simulink model "rf_thickener_open_loop"  (R2017a)
settings: Solver=VariableStepAuto  StartTime=0.0  StopTime=simTime  RelTol=1e-3  EnableMultiTasking=on
values from neighbouring files (symbols this model uses):
  addICInSimulation = zeros(1,5)    [OLD_compare_rf_thickener.m]    (also in OLD_compare_rf_thickener_PRBS.m; bogey.m = ones(1,5); compare_predictors.m = ones(1,5); compare_rf_thickener_RealData.m = ones(1,5))
  D0 = [325.1 0.3143 0.356]    [OLD_compare_rf_thickener.m]    (also in OLD_compare_rf_thickener_PRBS.m = [326.419 0.3 0.356]; bogey.m = [326.3733 0.3143 0.356]; compare_predictors.m = [326.3733 0.3143 0.356]; compare_rf_thickener_RealData.m = [326.3733 0.3143 0.356])
  Dt = 1    [OLD_compare_rf_thickener.m]    (also in OLD_compare_rf_thickener_PRBS.m; bogey.m; compare_predictors.m; compare_rf_thickener_RealData.m)
  m = length(MachineLearningData.MV)    [compare_predictors.m]    (also in compare_rf_thickener_RealData.m)
  make = makeMatrix(m,:)    [OLD_compare_rf_thickener.m]    (also in OLD_compare_rf_thickener_PRBS.m = makeMatrix(iterationSim,:); bogey.m = makeMatrix(iterationsSim,:); compare_predictors.m = makeStepMatrix(simIter,:); compare_rf_thickener_RealData.m = makeStepMatrix(simIter,:))
  nPredictors = [10 10 9 9]    [OLD_compare_rf_thickener.m]    (also in OLD_compare_rf_thickener_PRBS.m = [10 10 10 10])
  nTrees = [100 100 100 100]    [OLD_compare_rf_thickener.m]    (also in OLD_compare_rf_thickener_PRBS.m)
  tau_R = 10*groupBy    (= 600)    [OLD_compare_rf_thickener.m]    (also in OLD_compare_rf_thickener_PRBS.m = 300; bogey.m = 300; compare_predictors.m = 5; compare_rf_thickener_RealData.m = 300)
  U0 = [111 26]    [OLD_compare_rf_thickener.m]    (also in OLD_compare_rf_thickener_PRBS.m = [113.8675 25.715]; bogey.m = [114.8275 26.0152]; compare_predictors.m = [114.8275 26.0152]; compare_rf_thickener_RealData.m = [114.8275 26.0152])
undefined symbols (not defined in the file or in its folder): A, a1, a2, a3, B, b0, b1, b2, b3, b4, c0, c1, Cdata, Cz, Ddata, DiscIntNeverNeededParam, Dz, jf, kappa, L, lambda, mu, N, n_rz, na, nb, nc, phi0, phi_c, phi_f, rho_f, rho_s, theta, u10, u20, u30, v_max, w0, y, Z
settings Model: ExtModeTrigDuration=100  Creator=pablo  LastModifiedBy=Felipe
settings DataIOCC: SaveOutput=off  StateSaveName=tmp_raccel_xout  SignalLoggingName=tmp_raccel_logsout
settings OptimizationCC: EfficientMapNaN2IntZero=off  LifeSpan=inf
settings DebuggingCC: SFUnexpectedBacktrackingDiag=warning  SFNoUnconditionalDefaultTransitionDiag=warning  SFExecutionAtInitializationDiag=none
settings HardwareCC: TargetBitPerPointer=64  TargetBitPerSizeT=64  TargetBitPerPtrDiffT=64  TargetLongLongMode=on  TargetIntDivRoundTo=Zero  TargetEndianess=LittleEndian  TargetWordSize=64  TargetHWDeviceType=MATLAB Host  ProdEqTarget=off
settings RTWCC: SystemTargetFile=raccel.tlc  TemplateMakefile=raccel_default_tmf  RTWVerbose=off  RTWUseSimCustomCode=on
settings CodeAppCC: GenerateComments=off  MaxIdLength=128  MangleLength=10  SimulinkBlockComments=off
settings RaccelTargetCC: GeneratePreprocessorConditionals=Use local settings  ERTFirstTimeCompliant=off  MultiInstanceERTCode=off  ENABLE_SLEXEC_SSBRIDGE=0  RTWCAPIParams=on
settings ConfigComp: CovMetricSettings=dw  CovHtmlReporting=on  CovSaveCumulativeToWorkspaceVar=on  CovSaveSingleToWorkspaceVar=on  CovExternalEMLEnable=off

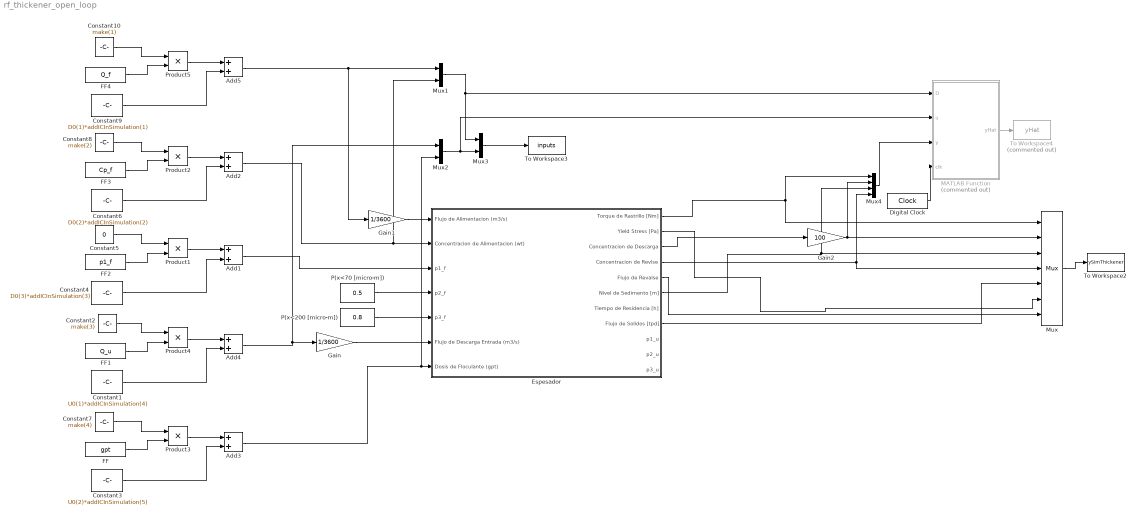
== system rf_thickener_open_loop ==
  Add{1..5} (5 alike) : Sum
  Constant1 : Constant  Value=U0(1)*addICInSimulation(4)
  Constant10 : Constant  Value=make(1)
  Constant2 : Constant  Value=make(3)
  Constant3 : Constant  Value=U0(2)*addICInSimulation(5)
  Constant4 : Constant  Value=D0(3)*addICInSimulation(3)
  Constant5 : Constant  Value=0
  Constant6 : Constant  Value=D0(2)*addICInSimulation(2)
  Constant7 : Constant  Value=make(4)
  Constant8 : Constant  Value=make(2)
  Constant9 : Constant  Value=D0(1)*addICInSimulation(1)
  Digital Clock : DigitalClock
  Espesador : Subsystem
  FF : FromWorkspace  VariableName=gpt  SampleTime=Dt
  FF1 : FromWorkspace  VariableName=Q_u  SampleTime=Dt
  FF2 : FromWorkspace  VariableName=p1_f  SampleTime=Dt
  FF3 : FromWorkspace  VariableName=Cp_f  SampleTime=Dt
  FF4 : FromWorkspace  VariableName=Q_f  SampleTime=Dt
  Gain : Gain  Gain=1/3600
  Gain1 : Gain  Gain=1/3600
  Gain2 : Gain  Gain=100
  MATLAB Function : MATLAB Function  Commented=on  TreatAsAtomicUnit=on
  Mux : Mux  Inputs=7
  Mux1 : Mux  Inputs=2
  Mux2 : Mux  Inputs=2
  Mux3 : Mux  Inputs=2
  Mux4 : Mux
  P(x<200 [micro-m]) : Constant  Value=0.8
  P(x<70 [micro-m]) : Constant  Value=0.5
  Product{1..5} (5 alike) : Product
  To Workspace2 : ToWorkspace  VariableName=ySimThickener  SaveFormat=Structure With Time  SampleTime=-1
  To Workspace3 : ToWorkspace  VariableName=inputs  SaveFormat=Structure With Time  SampleTime=-1
  To Workspace4 : ToWorkspace  Commented=on  VariableName=yHat  SaveFormat=Structure With Time  SampleTime=-1
  wires:
  P(x<200 [micro-m])/1 -> Espesador/5(p3_f)
  P(x<70 [micro-m])/1 -> Espesador/4(p2_f)
  FF/1 -> Product3/2
  Gain/1 -> Espesador/6(Flujo de Descarga Entrada (m3/s))
  Espesador/8(Flujo de Solidos [tpd]) -> Mux/5
  Espesador/2(Yield Stress [Pa]) -> Mux/6
  Espesador/5(Flujo de Revalse) -> Mux/7
  Mux/1 -> To Workspace2/1
  Constant7/1 -> Product3/1
  Product3/1 -> Add3/1
  Constant3/1 -> Add3/2
  Add3/1 -> Mux2/2, Espesador/7(Dosis de Floculante (gpt))
  Product4/1 -> Add4/1
  FF1/1 -> Product4/2
  Constant1/1 -> Add4/2
  Constant2/1 -> Product4/1
  Product1/1 -> Add1/1
  FF2/1 -> Product1/2
  Add1/1 -> Espesador/3(p1_f)
  Constant4/1 -> Add1/2
  Constant5/1 -> Product1/1
  Product2/1 -> Add2/1
  FF3/1 -> Product2/2
  Add2/1 -> Mux1/2, Espesador/2(Concentracion de Alimentacion (wt))
  Constant6/1 -> Add2/2
  Constant8/1 -> Product2/1
  Product5/1 -> Add5/1
  Constant10/1 -> Product5/1
  FF4/1 -> Product5/2
  Add5/1 -> Mux1/1, Gain1/1
  Constant9/1 -> Add5/2
  Add4/1 -> Mux2/1, Gain/1
  Mux3/1 -> To Workspace3/1
  Mux2/1 -> MATLAB Function/2(u), Mux3/2
  Mux1/1 -> Mux3/1, MATLAB Function/1(D)
  Digital Clock/1 -> MATLAB Function/4(clk)
  Mux4/1 -> MATLAB Function/3(y)
  MATLAB Function/1(yHat) -> To Workspace4/1
  Gain1/1 -> Espesador/1(Flujo de Alimentacion (m3/s))
  Espesador/1(Torque de Rastrillo [Nm]) -> Mux4/1, Mux/1
  Espesador/6(Nivel de Sedimento [m]) -> Mux/3, Mux4/3
  Espesador/4(Concentracion de Revlse) -> Mux/4, Mux4/4
  Espesador/3(Concentracion de Descarga) -> Gain2/1
  Gain2/1 -> Mux4/2, Mux/2

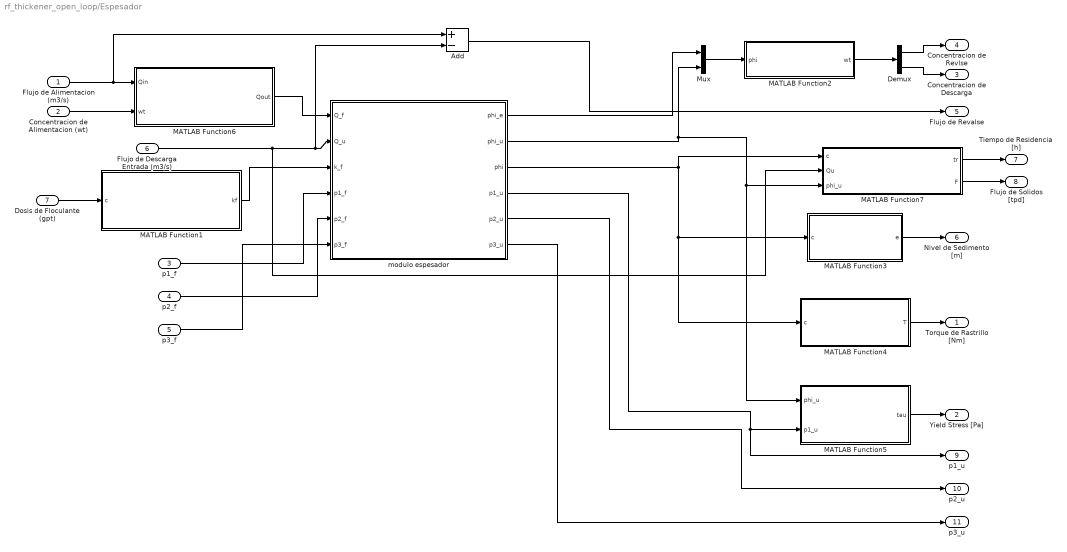
== system rf_thickener_open_loop/Espesador ==
  Flujo de Alimentacion (m3/s) : Inport
  Concentracion de Alimentacion (wt) : Inport  Port=2
  p1_f : Inport  Port=3
  p2_f : Inport  Port=4
  p3_f : Inport  Port=5
  Flujo de Descarga Entrada (m3/s) : Inport  Port=6
  Dosis de Floculante (gpt) : Inport  Port=7
  Add : Sum  Inputs=+-
  Demux : Demux  Outputs=2
  MATLAB Function1 : MATLAB Function  TreatAsAtomicUnit=on
  MATLAB Function2 : MATLAB Function  TreatAsAtomicUnit=on
  MATLAB Function3 : MATLAB Function  TreatAsAtomicUnit=on
  MATLAB Function4 : MATLAB Function  TreatAsAtomicUnit=on
  MATLAB Function5 : MATLAB Function  TreatAsAtomicUnit=on
  MATLAB Function6 : MATLAB Function  TreatAsAtomicUnit=on
  MATLAB Function7 : MATLAB Function  TreatAsAtomicUnit=on
  Mux : Mux  Inputs=2
  modulo espesador : Subsystem
  Torque de Rastrillo [Nm] : Outport
  Yield Stress [Pa] : Outport  Port=2
  Concentracion de Descarga : Outport  Port=3
  Concentracion de Revlse : Outport  Port=4
  Flujo de Revalse : Outport  Port=5
  Nivel de Sedimento [m] : Outport  Port=6
  Tiempo de Residencia [h] : Outport  Port=7
  Flujo de Solidos [tpd] : Outport  Port=8
  "p1_u " : Outport  Port=9
  "p2_u " : Outport  Port=10
  p3_u : Outport  Port=11
  wires:
  MATLAB Function3/1(e) -> Nivel de Sedimento [m]/1
  MATLAB Function4/1(T) -> Torque de Rastrillo [Nm]/1
  MATLAB Function5/1(tau) -> Yield Stress [Pa]/1
  Dosis de Floculante (gpt)/1 -> MATLAB Function1/1(c)
  Flujo de Descarga Entrada (m3/s)/1 -> MATLAB Function7/2(Qu), Add/2, modulo espesador/2(Q_u)
  MATLAB Function1/1(kf) -> modulo espesador/3(k_f)
  modulo espesador/1(phi_e) -> Mux/1
  modulo espesador/2(phi_u) -> MATLAB Function7/3(phi_u), MATLAB Function5/1(phi_u), Mux/2
  modulo espesador/5(p2_u) -> "p2_u "/1
  modulo espesador/3(phi) -> MATLAB Function7/1(c), MATLAB Function3/1(c), MATLAB Function4/1(c)
  p1_f/1 -> modulo espesador/4(p1_f)
  p2_f/1 -> modulo espesador/5("p2_f ")
  modulo espesador/4(p1_u) -> "p1_u "/1, MATLAB Function5/2(p1_u)
  Mux/1 -> MATLAB Function2/1(phi)
  MATLAB Function2/1(wt) -> Demux/1
  Demux/1 -> Concentracion de Revlse/1
  Demux/2 -> Concentracion de Descarga/1
  p3_f/1 -> modulo espesador/6(p3_f)
  modulo espesador/6(p3_u) -> p3_u/1
  MATLAB Function6/1(Qout) -> modulo espesador/1(Q_f)
  Flujo de Alimentacion (m3/s)/1 -> Add/1, MATLAB Function6/1(Qin)
  Concentracion de Alimentacion (wt)/1 -> MATLAB Function6/2(wt)
  MATLAB Function7/1(tr) -> Tiempo de Residencia [h]/1
  MATLAB Function7/2(F) -> Flujo de Solidos [tpd]/1
  Add/1 -> Flujo de Revalse/1

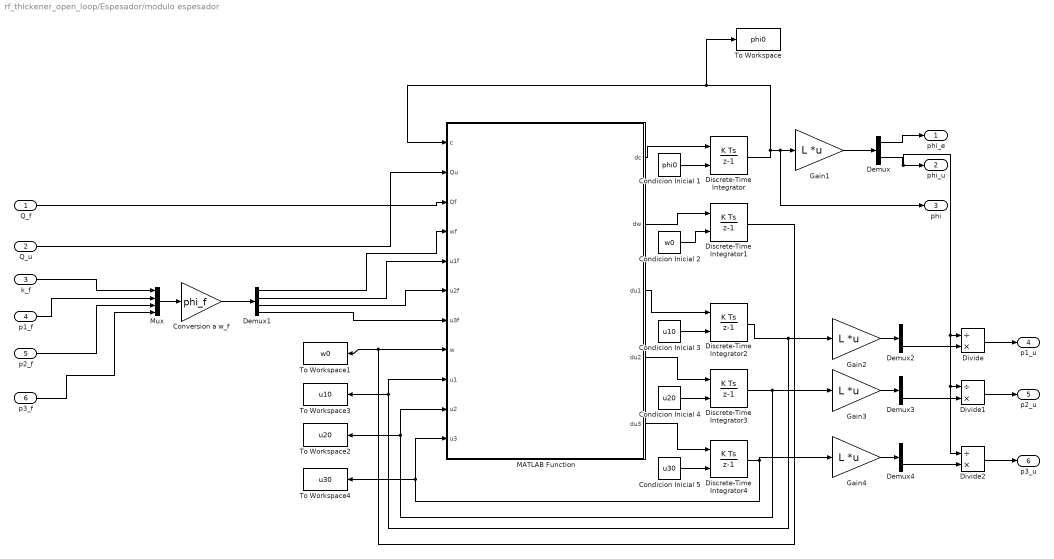
== system rf_thickener_open_loop/Espesador/modulo espesador ==
  Q_f : Inport
  Q_u : Inport  Port=2
  k_f : Inport  Port=3
  p1_f : Inport  Port=4
  "p2_f " : Inport  Port=5
  p3_f : Inport  Port=6
  Condicion Inicial 1 : Constant  Value=phi0
  Condicion Inicial 2 : Constant  Value=w0
  Condicion Inicial 3 : Constant  Value=u10
  Condicion Inicial 4 : Constant  Value=u20
  Condicion Inicial 5 : Constant  Value=u30
  Conversion a w_f : Gain  Gain=phi_f
  Demux{,2..4} (4 alike) : Demux  Outputs=2
  Demux1 : Demux
  Discrete-Time Integrator{,1..4} (5 alike) : DiscreteIntegrator  InitialConditionSource=external  InitialConditionSetting=State (most efficient)  SampleTime=Dt  ICPrevOutput=DiscIntNeverNeededParam  ICPrevScaledInput=DiscIntNeverNeededParam
  Divide : Product  Inputs=/*
  Divide1 : Product  Inputs=/*
  Divide2 : Product  Inputs=/*
  Gain{1..4} (4 alike) : Gain  Gain=L  Multiplication=Matrix(K*u) (u vector)
  MATLAB Function : MATLAB Function  TreatAsAtomicUnit=on
  Mux : Mux
  To Workspace : ToWorkspace  VariableName=phi0  SampleTime=-1
      settings: MaxDataPoints=1
  To Workspace1 : ToWorkspace  VariableName=w0  SampleTime=-1
      settings: MaxDataPoints=1
  To Workspace2 : ToWorkspace  VariableName=u20  SampleTime=-1
      settings: MaxDataPoints=1
  To Workspace3 : ToWorkspace  VariableName=u10  SampleTime=-1
      settings: MaxDataPoints=1
  To Workspace4 : ToWorkspace  VariableName=u30  SampleTime=-1
      settings: MaxDataPoints=1
  phi_e : Outport
  phi_u : Outport  Port=2
  phi : Outport  Port=3
  p1_u : Outport  Port=4
  p2_u : Outport  Port=5
  p3_u : Outport  Port=6
  wires:
  Discrete-Time Integrator/1 -> MATLAB Function/1(c), To Workspace/1, phi/1, Gain1/1
  Gain1/1 -> Demux/1
  Demux/1 -> phi_e/1
  Demux/2 -> Divide2/1, Divide1/1, Divide/1, phi_u/1
  MATLAB Function/1(dc) -> Discrete-Time Integrator/1
  Condicion Inicial 1/1 -> Discrete-Time Integrator/2
  Condicion Inicial 2/1 -> Discrete-Time Integrator1/2
  MATLAB Function/2(dw) -> Discrete-Time Integrator1/1
  Discrete-Time Integrator1/1 -> MATLAB Function/8(w), To Workspace1/1
  Q_f/1 -> MATLAB Function/3(Qf)
  Q_u/1 -> MATLAB Function/2(Qu)
  "p2_f "/1 -> Mux/3
  Mux/1 -> Conversion a w_f/1
  Conversion a w_f/1 -> Demux1/1
  Demux1/1 -> MATLAB Function/4(wf)
  Demux1/2 -> MATLAB Function/5(u1f)
  Demux1/3 -> MATLAB Function/6(u2f)
  Demux1/4 -> MATLAB Function/7(u3f)
  p3_f/1 -> Mux/4
  p1_f/1 -> Mux/2
  k_f/1 -> Mux/1
  Condicion Inicial 5/1 -> Discrete-Time Integrator4/2
  Condicion Inicial 4/1 -> Discrete-Time Integrator3/2
  MATLAB Function/5(du3) -> Discrete-Time Integrator4/1
  Discrete-Time Integrator4/1 -> To Workspace4/1, MATLAB Function/11(u3), Gain4/1
  MATLAB Function/4(du2) -> Discrete-Time Integrator3/1
  Discrete-Time Integrator3/1 -> Gain3/1, To Workspace2/1, MATLAB Function/10(u2)
  Condicion Inicial 3/1 -> Discrete-Time Integrator2/2
  MATLAB Function/3(du1) -> Discrete-Time Integrator2/1
  Discrete-Time Integrator2/1 -> Gain2/1, MATLAB Function/9(u1), To Workspace3/1
  Gain2/1 -> Demux2/1
  Demux2/2 -> Divide/2
  Divide/1 -> p1_u/1
  Gain3/1 -> Demux3/1
  Gain4/1 -> Demux4/1
  Divide1/1 -> p2_u/1
  Divide2/1 -> p3_u/1
  Demux3/2 -> Divide1/2
  Demux4/2 -> Divide2/2

== matlab function rf_thickener_open_loop/Espesador/MATLAB Function1 ==
  data: c input size=1; b0 parameter size=1; b1 parameter; kf output size=1; b2 parameter; b3 parameter; b4 parameter; v_max parameter
function kf = modelo_floculacion(c, b0, b1, b2, b3, b4, v_max)%#codegen

v = (b0+b1*(b2-c).*exp(-(c-b3).^2/b4))/3600;
kf = v/v_max;

== matlab function rf_thickener_open_loop/Espesador/modulo espesador/MATLAB Function ==
  data: c input size=N+3; Qu input size=1; Qf input size=1; wf input size=1; dc output size=N+3 [0..1]; dw output size=N+3; v_max parameter; n_rz parameter; lambda parameter; mu parameter; y parameter; jf parameter; N parameter; Dt parameter; Cdata parameter; Ddata parameter; phi_f parameter size=1; u1f input; u2f input; u3f input; w input size=N+3 [0..1]; du1 output; du2 output; du3 output; u1 input size=N+3; u2 input size=N+3; u3 input size=N+3
function [ dc, dw, du1, du2, du3] = modelo_espesador( c, Qu, Qf, wf, v_max, n_rz, lambda, mu, y, jf, N, Dt, Cdata, Ddata, phi_f, u1f, u2f, u3f, w, u1, u2, u3)%#codegen
%Metodo Numerico:
% "Modeling and controlling clarifier-thickeners fed by suspensions with
% time dependant properties" - Betancourt et al. 2014

%Variables Entrada:
% c = solid volume fraction j=-1...N+1
% w = conserved quantity j=-1...N+1
% cf = feed solid volume fraction (scalar)
% wf = feed value of conserved quantity (scalar)
% Qf = feed volume flow (m3/s)
% Qu = under-flow volume flow (m3/s)

%Variables de Salida:
% c = solid volume fraction j=-1...N+1
% w = conserved quantity j=-1...N+1
% Qe = effluent-flow volume flow (m3/s)
% cu = solid volume fraction of under-flow
% ce = solid volume fraction of effluent-flow

Qe = Qf - Qu;

assert (N < 1000);
assert (jf < 1000);

q = zeros(N+4,1);
dc1 = zeros(N+3,1);
dw1 = zeros(N+3,1);
du11 = zeros(N+3,1);
du21 = zeros(N+3,1);
du31 = zeros(N+3,1);
q(1:jf+2) = -Qe;
q(jf+3:end) = Qu;

%First step: linear contributions of the flux
dc1(1:jf+1) = - lambda(1:jf+1).*(q(2:jf+2).*(c(2:jf+2)-phi_f)-q(1:jf+1).*(c(1:jf+1)-phi_f));
dc1(jf+2) = - lambda(jf+2).*(q(jf+3).*(c(jf+2)-phi_f)-q(jf+2).*(c(jf+2)-phi_f));
dc1(jf+3:end) = - lambda(jf+3:end).*(q(jf+4:end).*(c(jf+3:end)-phi_f)-q(jf+3:end-1).*(c(jf+2:end-1)-phi_f));

c1 = c + Dt*dc1;

D = numerical_compression_flux(c1,Ddata,Cdata);
Dp = [D(2:end); 0]; Dm = [0; D(1:end-1)];

dw1(1:jf+1) = - lambda(1:jf+1).*(q(2:jf+2).*(w(2:jf+2)-wf)-q(1:jf+1).*(w(1:jf+1)-wf));
dw1(jf+2) = - lambda(jf+2).*(q(jf+3).*(w(jf+2)-wf)-q(jf+2).*(w(jf+2)-wf));
dw1(jf+3:end) = - lambda(jf+3:end).*(q(jf+4:end).*(w(jf+3:end)-wf)-q(jf+3:end-1).*(w(jf+2:end-1)-wf));

w1 = w + Dt*dw1;

du11(1:jf+1) = - lambda(1:jf+1).*(q(2:jf+2).*(u1(2:jf+2)-u1f)-q(1:jf+1).*(u1(1:jf+1)-u1f));
du11(jf+2) = - lambda(jf+2).*(q(jf+3).*(u1(jf+2)-u1f)-q(jf+2).*(u1(jf+2)-u1f));
du11(jf+3:end) = - lambda(jf+3:end).*(q(jf+4:end).*(u1(jf+3:end)-u1f)-q(jf+3:end-1).*(u1(jf+2:end-1)-u1f));

u11 = u1 + Dt*du11;

du21(1:jf+1) = - lambda(1:jf+1).*(q(2:jf+2).*(u2(2:jf+2)-u2f)-q(1:jf+1).*(u2(1:jf+1)-u2f));
du21(jf+2) = - lambda(jf+2).*(q(jf+3).*(u2(jf+2)-u2f)-q(jf+2).*(u2(jf+2)-u2f));
du21(jf+3:end) = - lambda(jf+3:end).*(q(jf+4:end).*(u2(jf+3:end)-u2f)-q(jf+3:end-1).*(u2(jf+2:end-1)-u2f));

u21 = u2 + Dt*du21;

du31(1:jf+1) = - lambda(1:jf+1).*(q(2:jf+2).*(u3(2:jf+2)-u3f)-q(1:jf+1).*(u3(1:jf+1)-u3f));
du31(jf+2) = - lambda(jf+2).*(q(jf+3).*(u3(jf+2)-u3f)-q(jf+2).*(u3(jf+2)-u3f));
du31(jf+3:end) = - lambda(jf+3:end).*(q(jf+4:end).*(u3(jf+3:end)-u3f)-q(jf+3:end-1).*(u3(jf+2:end-1)-u3f));

u31 = u3 + Dt*du31;

%Variable computation
k=c1; k(c1>eps)=w1(c1>eps)./c1(c1>eps);

V=y(3:N+2).*k(3:N+2).*v_hs(c1(3:N+2),v_max,n_rz); Vp = [0; V; 0; 0]; Vm = [0; 0; V; 0];

k1 = (c1(2:N+1)>=c1(3:N+2)).*k(2:N+1) + (c1(2:N+1)<c1(3:N+2)).*k(3:N+2); k1p = [0; k1; 0; 0]; k1m = [0; 0; k1; 0];

w2 = (c1(2:N+1)>=c1(3:N+2)).*w1(2:N+1) + (c1(2:N+1)<c1(3:N+2)).*w1(3:N+2); w2p = [0; w2; 0; 0]; w2m = [0; 0; w2; 0];

u12 = (c1(2:N+1)>=c1(3:N+2)).*u11(2:N+1) + (c1(2:N+1)<c1(3:N+2)).*u11(3:N+2); u12p = [0; u12; 0; 0]; u12m = [0; 0; u12; 0];

u22 = (c1(2:N+1)>=c1(3:N+2)).*u21(2:N+1) + (c1(2:N+1)<c1(3:N+2)).*u21(3:N+2); u22p = [0; u22; 0; 0]; u22m = [0; 0; u22; 0];

u32 = (c1(2:N+1)>=c1(3:N+2)).*u31(2:N+1) + (c1(2:N+1)<c1(3:N+2)).*u31(3:N+2); u32p = [0; u32; 0; 0]; u32m = [0; 0; u32; 0];

yp = y(2:N+4); ym = y(1:N+3);

c1m = [0; c1(1:end-1)];
w1m = [0; w1(1:end-1)];
u11m = [0; u11(1:end-1)];
u21m = [0; u21(1:end-1)];
u31m = [0; u31(1:end-1)];

%Second step: non-linear contributions of the flux

dc = dc1 - lambda.*(Vp.*c1-Vm.*c1m) + mu.*(yp.*w2p.*(Dp-D)-ym.*w2m.*(D-Dm));
dw = dw1 - lambda.*(Vp.*w1-Vm.*w1m) + mu.*(yp.*w2p.*k1p.*(Dp-D)-ym.*w2m.*k1m.*(D-Dm));
du1 = du11 - lambda.*(Vp.*u11-Vm.*u11m) + mu.*(yp.*u12p.*k1p.*(Dp-D)-ym.*u12m.*k1m.*(D-Dm));
du2 = du21 - lambda.*(Vp.*u21-Vm.*u21m) + mu.*(yp.*u22p.*k1p.*(Dp-D)-ym.*u22m.*k1m.*(D-Dm));
du3 = du31 - lambda.*(Vp.*u31-Vm.*u31m) + mu.*(yp.*u32p.*k1p.*(Dp-D)-ym.*u32m.*k1m.*(D-Dm));

== matlab function rf_thickener_open_loop/Espesador/MATLAB Function2 ==
  data: phi input; wt output; rho_s parameter; rho_f parameter
function wt = volume_to_weight_fraction(phi, rho_s, rho_f)
%#codegen

wt = phi*rho_s./(phi*rho_s+(1-phi)*rho_f);

== matlab function rf_thickener_open_loop/Espesador/MATLAB Function3 ==
  data: c input; e output; phi_c parameter; Z parameter size=N+3; B parameter
function e = modelo_nivel_sedimento(c, phi_c, Z, B)%#codegen

if (sum(c>=phi_c)>=2)
    % If two or more layers exhibit concentration greater than phi_c, then
    % there is a sedimentation layer.
    e = min(Z(c>=phi_c));
    % The height of the sedimentation layer is measured from feedwell (z =
    % 0) to bottom (z = 12). The above command returns the minimum of the Z
    % that has a phi >= phi_c. Therefore, it returns the height measured
    % from the feedwell to the critical interphase. Therefore, it measures
    % the width of the interphase region.
    % The thickness of the sedimentation layer (from the bottom of the
    % thickener) is B-e.
else
    e = B;
end

== matlab function rf_thickener_open_loop/Espesador/MATLAB Function4 ==
  data: c input; T output; Cz parameter; a1 parameter; a2 parameter; a3 parameter
function T = modelo_torque_rastrillo(c,Cz,a1,a2,a3)
%#codegen

T = a1*(Cz'*c).^a2+a3;

== matlab function rf_thickener_open_loop/Espesador/MATLAB Function5 ==
  data: phi_u input; p1_u input; tau output; kappa parameter; m parameter; rho_s parameter; c0 parameter; c1 parameter; theta parameter; rho_f parameter
function tau = modelo_yield_stress(phi_u,p1_u,kappa,m,rho_s, c0,c1,theta, rho_f)
%#codegen

    rho = c0 + c1*(p1_u-theta).^2;
    wt = phi_u*rho_s./(phi_u*rho_s+(1-phi_u)*rho_f);
    Sr = rho.*rho_s./(rho_s-rho).*(1-wt)*1e-3;
    tau = kappa*Sr.^(-m);

== matlab function rf_thickener_open_loop/Espesador/MATLAB Function6 ==
  data: Qin input size=1; phi_f parameter; Qout output size=1; wt input size=1; rho_f parameter; rho_s parameter
function Qout = modelo_dilucion(Qin,phi_f, wt,rho_f, rho_s)%#codegen

phi = (wt*rho_f)/(wt*rho_f+(1-wt)*rho_s);

Qout = Qin*phi/phi_f;

== matlab function rf_thickener_open_loop/Espesador/MATLAB Function7 ==
  data: c input size=N+3; tr output; A parameter size=N+3; Dz parameter; F output; rho_s parameter; Qu input; phi_u input
function [tr, F] = modelo_tiempo_de_residencia(c, A, Dz, rho_s, Qu, phi_u)%#codegen

F = Qu*phi_u; %m3/s de solido
tr = (A'*c)*Dz/F/3600; %h
F = F*rho_s*3.6*24; %tpd de solido

end

== matlab function rf_thickener_open_loop/MATLAB Function ==
  data: D input; yHat output size=[4 1]; u input; y input; clk input; nTrees parameter; nPredictors parameter; na parameter; nb parameter; nc parameter; yPastValues data_store_memory; uPastValues data_store_memory; dPastValues data_store_memory; tau_R parameter
function yHat = rf_plant_model(D, u, y, clk,...
                nTrees, nPredictors, na, nb, nc,tau_R)
coder.extrinsic('predictRF_Y1_mex');
coder.extrinsic('predictRF_Y2_mex');
coder.extrinsic('predictRF_Y3_mex');
coder.extrinsic('predictRF_Y4_mex');
% coder.extrinsic('predictRF_Y1_PRBS_mex');
% coder.extrinsic('predictRF_Y2_PRBS_mex');
% coder.extrinsic('predictRF_Y3_PRBS_mex');
% coder.extrinsic('predictRF_Y4_PRBS_mex');

global yPastValues
global uPastValues
global dPastValues


%   - nc: n*d containing order of DV delay for each CV
[n,~] = size(na);
[n,m] = size(nb);
[n,d] = size(nc);
yHat = zeros(n,1);
if rem(clk,tau_R) == 0
    

    predictorArray = generate_predictor_array_OL(yPastValues,uPastValues,dPastValues,...
                                                na,nb,nc);
    for cv = 1:n
        % Predict
    %     p = na(cv)+sum(nb(cv,:))+m+nc(cv,:)+d;
        p = na(cv)+sum(nb(cv,:))+sum(nc(cv,:));
        if nTrees(cv) ~= 100
           error('Number of trees is %d in hardcoded function. Different from: %d',100,nTrees(cv)); 
        end
        if nPredictors(cv) ~= p
           error('Number of predictors is %d in hardcoded function. Different from: %d',p,nPredictors(cv)); 
        end
        X = predictorArray(cv,1:p);
        switch cv
            case 1
                yHat(cv,1) = predictRF_Y1_mex(X,nTrees(cv),p);
            case 2
                yHat(cv,1) = predictRF_Y2_mex(X,nTrees(cv),p);
            case 3
                yHat(cv,1) = predictRF_Y3_mex(X,nTrees(cv),p);
            case 4
                yHat(cv,1) = predictRF_Y4_mex(X,nTrees(cv),p);
        end
    end
    
    % Refresh past values for prediction in t+tau_R
    yPastValues(:,2:end) = yPastValues(:,1:end-1);
    yPastValues(:,1) = y(:);

    dPastValues(:,2:end) = dPastValues(:,1:end-1);
    dPastValues(:,1) = D(:);

    uPastValues(:,2:end) = uPastValues(:,1:end-1);
    uPastValues(:,1) = u(:);
end
